simulink model "half_step"  (R2021b)
settings: Solver=FixedStepDiscrete  StartTime=0.0  StopTime=inf  FixedStep=1e-4  RelTol=1e-3
libraries: simulink_extras x3, speedgoatlib_IO102 x2
settings Model: Creator=wasynczu  LastModifiedBy=wasynczu
settings SolverCC: ConcurrentTasks=on  PositivePriorityOrder=on
settings OptimizationCC: BlockReduction=off  OptimizeBlockIOStorage=off
settings DebuggingCC: TasksWithSamePriorityMsg=none
settings HardwareCC: ProdBitPerLong=64  ProdLongLongMode=on  ProdHWDeviceType=Intel->x86-64 (Linux 64)
settings RTWCC: Description=Simulink Real-Time  SystemTargetFile=slrealtime.tlc  TemplateMakefile=slrealtime_default_tmf  Toolchain=Simulink Real-Time Toolchain  BuildConfiguration=Faster Runs  CodeExecutionProfiling=on  TargetLang=C++

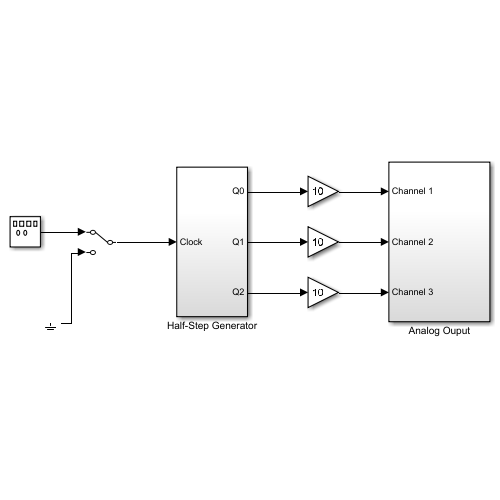
[thumbnail: Simulink's stored preview of the top-level diagram]
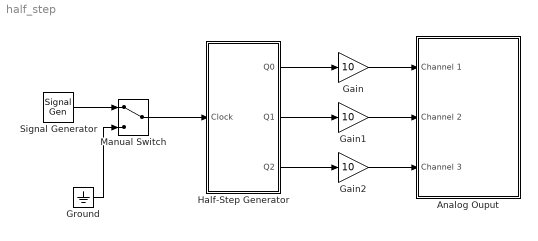
== system half_step ==
  Analog Ouput : Subsystem
  Gain : Gain  Gain=10
  Gain1 : Gain  Gain=10
  Gain2 : Gain  Gain=10
  Ground : Ground
  Half-Step Generator : Subsystem
  Manual Switch : ManualSwitch
  Signal Generator : SignalGenerator  WaveForm=square  Frequency=10
  wires:
  Manual Switch/1 -> Half-Step Generator/1(Clock)
  Signal Generator/1 -> Manual Switch/1
  Ground/1 -> Manual Switch/2
  Half-Step Generator/1(Q0) -> Gain/1
  Half-Step Generator/2(Q1) -> Gain1/1
  Half-Step Generator/3(Q2) -> Gain2/1
  Gain/1 -> Analog Ouput/1(Channel 1)
  Gain2/1 -> Analog Ouput/3(Channel 3)
  Gain1/1 -> Analog Ouput/2(Channel 2)

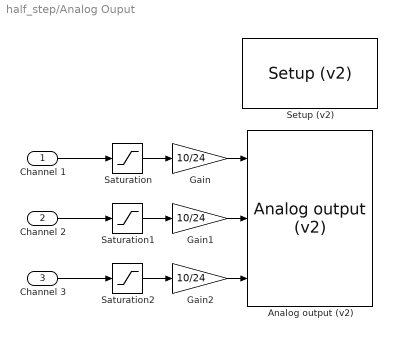
== system half_step/Analog Ouput ==
  Channel 1 : Inport
  Channel 2 : Inport  Port=2
  Channel 3 : Inport  Port=3
  "Analog output (v2) " : speedgoatlib_IO102/Analog output (v2)   id=1  channels=[1 2 3]  range=1  ts=-1  pciSlot=-1
      settings: SourceProductName=Simulink Real-Time: Speedgoat I/O Blockset
  Gain : Gain  Gain=10/24
  Gain1 : Gain  Gain=10/24
  Gain2 : Gain  Gain=10/24
  Saturation : Saturate  UpperLimit=24  LowerLimit=-24
  Saturation1 : Saturate  UpperLimit=24  LowerLimit=-24
  Saturation2 : Saturate  UpperLimit=24  LowerLimit=-24
  "Setup (v2) " : speedgoatlib_IO102/Setup (v2)   id=1  range=+-10V  cal=off  pciSlot=-1  adCoupling=Single-ended  adChannelMode=Multiple-channel (enter number of channels below)  adChannel=4  daChannel=[1,2,3]  daInitValue=[0]  daReset=[1]  DioDirectionLo=Input  DioDirectionHi=Output  doChannel=[9]  doInitValue=[0]  doReset=[1]  diChannel=[1]
      settings: SourceProductName=Simulink Real-Time: Speedgoat I/O Blockset
  wires:
  Saturation/1 -> Gain/1
  Saturation1/1 -> Gain1/1
  Saturation2/1 -> Gain2/1
  Gain1/1 -> "Analog output (v2) "/2
  Gain/1 -> "Analog output (v2) "/1
  Gain2/1 -> "Analog output (v2) "/3
  Channel 2/1 -> Saturation1/1
  Channel 3/1 -> Saturation2/1
  Channel 1/1 -> Saturation/1

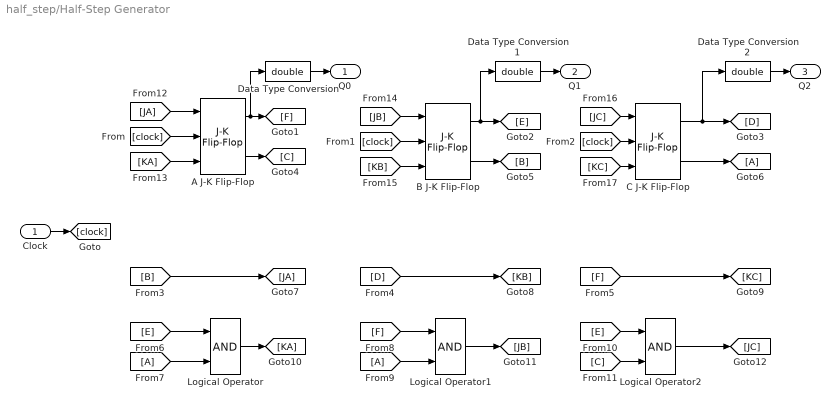
== system half_step/Half-Step Generator ==
  Clock : Inport
  A J-K Flip-Flop : simulink_extras/Flip Flops/J-K Flip-Flop  initial_condition=0
  B J-K Flip-Flop : simulink_extras/Flip Flops/J-K Flip-Flop  initial_condition=0
  C J-K Flip-Flop : simulink_extras/Flip Flops/J-K Flip-Flop  initial_condition=0
  Data Type Conversion : DataTypeConversion  OutDataTypeStr=double
  Data Type Conversion1 : DataTypeConversion  OutDataTypeStr=double
  Data Type Conversion2 : DataTypeConversion  OutDataTypeStr=double
  Logical Operator : Logic  AllPortsSameDT=off  OutDataTypeStr=boolean
  Logical Operator1 : Logic  AllPortsSameDT=off  OutDataTypeStr=boolean
  Logical Operator2 : Logic  AllPortsSameDT=off  OutDataTypeStr=boolean
  Q0 : Outport
  Q1 : Outport  Port=2
  Q2 : Outport  Port=3
  wires:
  Clock/1 -> [clock]
  [clock] -> A J-K Flip-Flop/2
  [clock] -> B J-K Flip-Flop/2
  [clock] -> C J-K Flip-Flop/2
  A J-K Flip-Flop/1 -> Data Type Conversion/1, [F]
  B J-K Flip-Flop/1 -> Data Type Conversion1/1, [E]
  C J-K Flip-Flop/1 -> Data Type Conversion2/1, [D]
  A J-K Flip-Flop/2 -> [C]
  B J-K Flip-Flop/2 -> [B]
  C J-K Flip-Flop/2 -> [A]
  [B] -> [JA]
  [D] -> [KB]
  [F] -> [KC]
  [E] -> Logical Operator/1
  [A] -> Logical Operator/2
  Logical Operator/1 -> [KA]
  [F] -> Logical Operator1/1
  [A] -> Logical Operator1/2
  Logical Operator1/1 -> [JB]
  [E] -> Logical Operator2/1
  [C] -> Logical Operator2/2
  Logical Operator2/1 -> [JC]
  [JA] -> A J-K Flip-Flop/1
  [KA] -> A J-K Flip-Flop/3
  [JB] -> B J-K Flip-Flop/1
  [KB] -> B J-K Flip-Flop/3
  [JC] -> C J-K Flip-Flop/1
  [KC] -> C J-K Flip-Flop/3
  Data Type Conversion/1 -> Q0/1
  Data Type Conversion1/1 -> Q1/1
  Data Type Conversion2/1 -> Q2/1
